simulink model "untitled"  (R2023a)
settings: Solver=VariableStepAuto  StartTime=0.0  StopTime=500  RelTol=1e-3
values from neighbouring files (symbols this model uses):
  d = 44.51e-3    (= 0.04451)    [Atv01.m]
  Ic = 130.7e-3    (= 0.1307)    [Atv01.m]
  Kb = 23e-3    (= 0.023)    [Atv01.m]
  Kt = 29e-3    (= 0.029)    [Atv01.m]
  L = 0.1655    [Atv01.m]
  La = 0.66e-3    (= 0.00066)    [Atv01.m]
  m = mc + 2*mw    (= 16)    [Atv01.m]
  N = 38.3    [Atv01.m]
  R = D/2    (= 0.0975)    [Atv01.m]
  Ra = 710e-3    (= 0.71)    [Atv01.m]
settings Model: Creator=Matheus  LastModifiedBy=Matheus

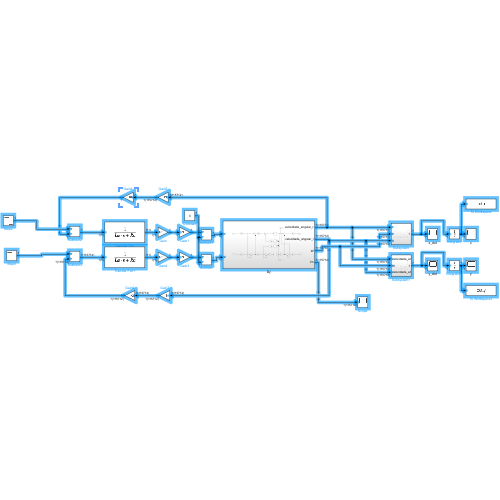
[thumbnail: Simulink's stored preview of the top-level diagram]
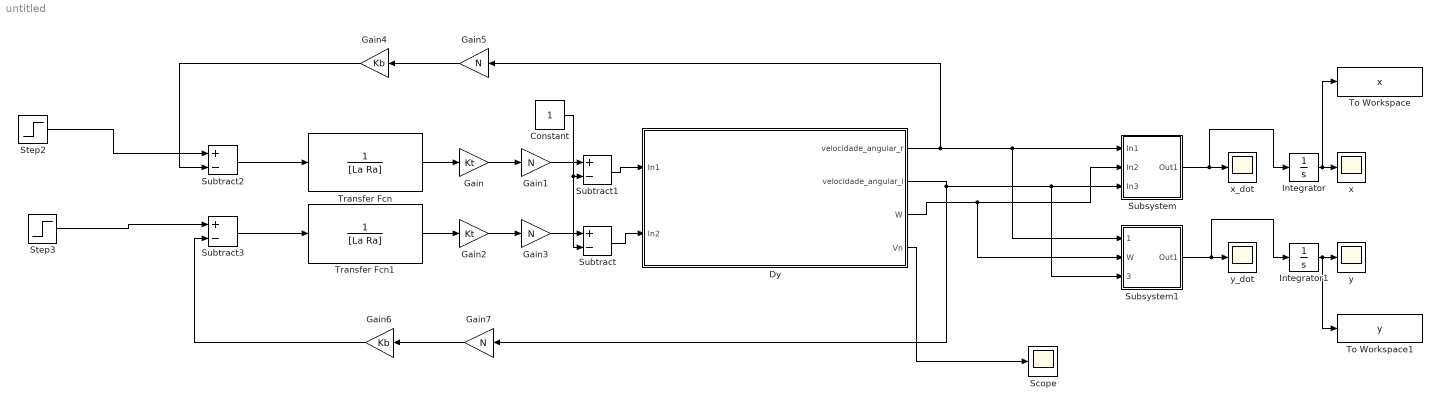
== system untitled ==
  Constant : Constant
  Dy : Subsystem
  Gain : Gain  Gain=Kt
  Gain{1,3,5,7} (4 alike) : Gain  Gain=N
  Gain2 : Gain  Gain=Kt
  Gain4 : Gain  Gain=Kb
  Gain6 : Gain  Gain=Kb
  Integrator : Integrator
  Integrator1 : Integrator
  Scope : Scope
  Step2 : Step  Before=10  After=5  SampleTime=0
  Step3 : Step  Before=10  After=8  SampleTime=0
  Subsystem : Subsystem
  Subsystem1 : Subsystem
  Subtract{,1..3} (4 alike) : Sum  Inputs=+-
  To Workspace : ToWorkspace  VariableName=x  SaveFormat=Structure With Time  SampleTime=-1
  To Workspace1 : ToWorkspace  VariableName=y  SaveFormat=Structure With Time  SampleTime=-1
  Transfer Fcn : TransferFcn  Denominator=[La Ra]
  Transfer Fcn1 : TransferFcn  Denominator=[La Ra]
  x : Scope
  x_dot : Scope
  y : Scope
  y_dot : Scope
  wires:
  Dy/1(velocidade_angular_r) -> Subsystem1/1(velocidade_angular_r), Subsystem/1(In1), Gain5/1
  Dy/2(velocidade_angular_l) -> Gain7/1, Subsystem1/3(velocidade_angular_l), Subsystem/3(In3)
  Gain3/1 -> Subtract/1
  Gain2/1 -> Gain3/1
  Transfer Fcn1/1 -> Gain2/1
  Transfer Fcn/1 -> Gain/1
  Gain/1 -> Gain1/1
  Gain1/1 -> Subtract1/1
  Subtract/1 -> Dy/2(In2)
  Subtract1/1 -> Dy/1(In1)
  Gain5/1 -> Gain4/1
  Subtract2/1 -> Transfer Fcn/1
  Gain4/1 -> Subtract2/2
  Gain7/1 -> Gain6/1
  Gain6/1 -> Subtract3/2
  Subtract3/1 -> Transfer Fcn1/1
  Dy/4(Vn) -> Scope/1
  Dy/3(W) -> Subsystem1/2(W), Subsystem/2(In2)
  Subsystem/1(Out1) -> Integrator/1, x_dot/1
  Subsystem1/1(Out1) -> Integrator1/1, y_dot/1
  Constant/1 -> Subtract/2, Subtract1/2
  Integrator/1 -> To Workspace/1, x/1
  Integrator1/1 -> To Workspace1/1, y/1
  Step2/1 -> Subtract2/1
  Step3/1 -> Subtract3/1

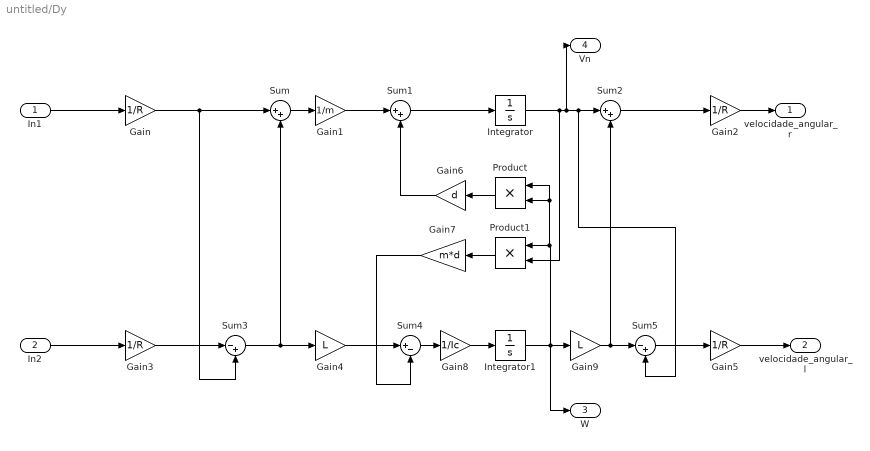
== system untitled/Dy ==
  In1 : Inport
  In2 : Inport  Port=2
  Gain{,2..3,5} (4 alike) : Gain  Gain=1/R
  Gain1 : Gain  Gain=1/m
  Gain4 : Gain  Gain=L
  Gain6 : Gain  Gain=d
  Gain7 : Gain  Gain=m*d
  Gain8 : Gain  Gain=1/Ic
  Gain9 : Gain  Gain=L
  Integrator : Integrator
  Integrator1 : Integrator
  Product : Product
  Product1 : Product
  Sum : Sum  Inputs=|++
  Sum1 : Sum  Inputs=|++
  Sum2 : Sum  Inputs=|++
  Sum3 : Sum  Inputs=|-+
  Sum4 : Sum  Inputs=|+-
  Sum5 : Sum  Inputs=|-+
  velocidade_angular_r : Outport
  velocidade_angular_l : Outport  Port=2
  W : Outport  Port=3
  Vn : Outport  Port=4
  wires:
  Sum5/1 -> Gain5/1
  Integrator/1 -> Product1/2, Vn/1, Sum2/1, Sum5/2
  Gain7/1 -> Sum4/2
  Integrator1/1 -> W/1, Gain9/1, Product/2, Product/1, Product1/1
  Sum3/1 -> Gain4/1, Sum/2
  Gain4/1 -> Sum4/1
  Sum/1 -> Gain1/1
  Gain3/1 -> Sum3/1
  Gain1/1 -> Sum1/1
  Sum2/1 -> Gain2/1
  Gain9/1 -> Sum5/1, Sum2/2
  Product1/1 -> Gain7/1
  Gain/1 -> Sum3/2, Sum/1
  In2/1 -> Gain3/1
  Sum1/1 -> Integrator/1
  Sum4/1 -> Gain8/1
  Gain8/1 -> Integrator1/1
  Product/1 -> Gain6/1
  Gain6/1 -> Sum1/2
  Gain2/1 -> velocidade_angular_r/1
  In1/1 -> Gain/1
  Gain5/1 -> velocidade_angular_l/1

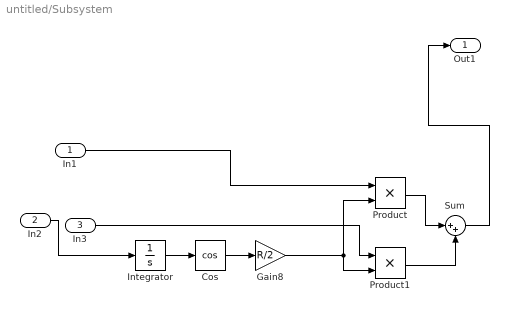
== system untitled/Subsystem ==
  In1 : Inport
  In2 : Inport  Port=2
  In3 : Inport  Port=3
  Cos : Trigonometry  Operator=cos
  Gain8 : Gain  Gain=R/2
  Integrator : Integrator
  Product : Product
  Product1 : Product
  Sum : Sum  Inputs=|++
  Out1 : Outport
  wires:
  In2/1 -> Integrator/1
  Cos/1 -> Gain8/1
  Product1/1 -> Sum/2
  Gain8/1 -> Product1/2, Product/2
  In1/1 -> Product/1
  Integrator/1 -> Cos/1
  Product/1 -> Sum/1
  Sum/1 -> Out1/1
  In3/1 -> Product1/1

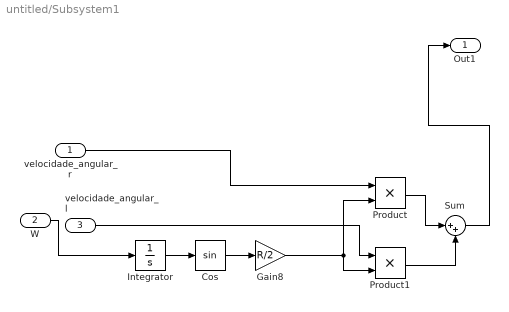
== system untitled/Subsystem1 ==
  velocidade_angular_r : Inport
  W : Inport  Port=2
  velocidade_angular_l : Inport  Port=3
  Cos : Trigonometry
  Gain8 : Gain  Gain=R/2
  Integrator : Integrator
  Product : Product
  Product1 : Product
  Sum : Sum  Inputs=|++
  Out1 : Outport
  wires:
  W/1 -> Integrator/1
  Cos/1 -> Gain8/1
  Product1/1 -> Sum/2
  Gain8/1 -> Product1/2, Product/2
  velocidade_angular_r/1 -> Product/1
  Integrator/1 -> Cos/1
  Product/1 -> Sum/1
  Sum/1 -> Out1/1
  velocidade_angular_l/1 -> Product1/1
